simulink model "Demo_veDYNA_cs"  (Simulink 7.6)
settings: Solver=ode1  SolverMode=SingleTasking  StartTime=0  StopTime=15  FixedStep=1/500  RelTol=1e-3
PreLoadFcn:
  | PreScanveDYNAPreLoadFcn(bdroot);
  | check_NUTS_defined;
  | 
  | assignin('base',['model_closed_' bdroot],false);
PostLoadFcn:
  | PreScanveDYNAPostLoadFcn(bdroot);
  | 
InitFcn:
  | vdy_SetExternalInputSource('ManLongCtrl',1,'Brake','other');
  | vdy_SetExternalInputSource('ManLongCtrl',1,'EngineTorque','other');
  | vdy_SetExternalInputSource('ManLatCtrl',1,'Steering','other');
  | 
  | PreScanveDYNAInitFcn(bdroot);
  | PreScanExperimentInitFcn(bdroot)
StopFcn:
  | PreScanExperimentStopFcn(bdroot)
undefined symbols (not defined in the file): at_period, CPT, DiscIntNeverNeededParam, vm_at_pulsewidth, vm_driver_dflt_gain, x_ini_VRML, y_ini_VRML, z_ini_VRML
libraries: dyna_cpt_lib x93, PreScanSimulinkLibrary x10, PreScanUsefulBlocks x4, simulink x4, anilib x3, dyna_lib x3, simulink_extras x2, dyna_manctrl_lib x2, dyna_road_lib x2, dyna_io_lib x1, dyna_demo_lib x1, dyna_usr_maneuver_states_lib x1
(part 7 of 8)

== system Demo_veDYNA_cs/Vedyna_Vehicle/CPT_MDL/MDL_PAR/ManLongCtrl/System Instance 1/AccelerationY [m/s**2] ==
  Table : Lookup  InputValues=CPT.MDL_PAR.ManLongCtrl{1}.AccelerationY.Table.x  Table=CPT.MDL_PAR.ManLongCtrl{1}.AccelerationY.Table.v  SaturateOnIntegerOverflow=on
  Terminator : Terminator
  Terminator1 : Terminator
  Value : Constant  Value=CPT.MDL_PAR.ManLongCtrl{1}.AccelerationY.Value.v
  tag scope: ManLongCtrl_1_AccelerationY_TBL=global, ManLongCtrl_1_AccelerationY_VAL=global
  wires:
  [vdy_Simctrl_tsim] -> Table/1
  Value/1 -> [ManLongCtrl_1_AccelerationY_VAL]
  [ManLongCtrl_1_AccelerationY_VAL] -> Terminator/1
  [ManLongCtrl_1_AccelerationY_TBL] -> Terminator1/1
  Table/1 -> [ManLongCtrl_1_AccelerationY_TBL]

== system Demo_veDYNA_cs/Vedyna_Vehicle/CPT_MDL/MDL_PAR/ManLongCtrl/System Instance 1/Brake [%] ==
  Table : Lookup  InputValues=CPT.MDL_PAR.ManLongCtrl{1}.Brake.Table.x  Table=CPT.MDL_PAR.ManLongCtrl{1}.Brake.Table.v  SaturateOnIntegerOverflow=on
  Terminator : Terminator
  Terminator1 : Terminator
  Value : Constant  Value=CPT.MDL_PAR.ManLongCtrl{1}.Brake.Value.v
  tag scope: ManLongCtrl_1_Brake_TBL=global, ManLongCtrl_1_Brake_VAL=global
  wires:
  [vdy_Simctrl_tsim] -> Table/1
  Value/1 -> [ManLongCtrl_1_Brake_VAL]
  [ManLongCtrl_1_Brake_VAL] -> Terminator/1
  [ManLongCtrl_1_Brake_TBL] -> Terminator1/1
  Table/1 -> [ManLongCtrl_1_Brake_TBL]

== system Demo_veDYNA_cs/Vedyna_Vehicle/CPT_MDL/MDL_PAR/ManLongCtrl/System Instance 1/EngineTorque [Nm] ==
  Table : Lookup  InputValues=CPT.MDL_PAR.ManLongCtrl{1}.EngineTorque.Table.x  Table=CPT.MDL_PAR.ManLongCtrl{1}.EngineTorque.Table.v  SaturateOnIntegerOverflow=on
  Terminator : Terminator
  Terminator1 : Terminator
  Value : Constant  Value=CPT.MDL_PAR.ManLongCtrl{1}.EngineTorque.Value.v
  tag scope: ManLongCtrl_1_EngineTorque_TBL=global, ManLongCtrl_1_EngineTorque_VAL=global
  wires:
  [vdy_Simctrl_tsim] -> Table/1
  Value/1 -> [ManLongCtrl_1_EngineTorque_VAL]
  [ManLongCtrl_1_EngineTorque_VAL] -> Terminator/1
  [ManLongCtrl_1_EngineTorque_TBL] -> Terminator1/1
  Table/1 -> [ManLongCtrl_1_EngineTorque_TBL]

== system Demo_veDYNA_cs/Vedyna_Vehicle/CPT_MDL/MDL_PAR/ManLongCtrl/System Instance 1/Speed [km/h] ==
  Table : Lookup  InputValues=CPT.MDL_PAR.ManLongCtrl{1}.Speed.Table.x  Table=CPT.MDL_PAR.ManLongCtrl{1}.Speed.Table.v  SaturateOnIntegerOverflow=on
  Terminator : Terminator
  Terminator1 : Terminator
  Value : Constant  Value=CPT.MDL_PAR.ManLongCtrl{1}.Speed.Value.v
  tag scope: ManLongCtrl_1_Speed_TBL=global, ManLongCtrl_1_Speed_VAL=global
  wires:
  [vdy_Simctrl_tsim] -> Table/1
  Value/1 -> [ManLongCtrl_1_Speed_VAL]
  [ManLongCtrl_1_Speed_VAL] -> Terminator/1
  [ManLongCtrl_1_Speed_TBL] -> Terminator1/1
  Table/1 -> [ManLongCtrl_1_Speed_TBL]

== system Demo_veDYNA_cs/Vedyna_Vehicle/CPT_MDL/MDL_PAR/ManLongCtrl/System Instance 1/Throttle [%] ==
  Table : Lookup  InputValues=CPT.MDL_PAR.ManLongCtrl{1}.Throttle.Table.x  Table=CPT.MDL_PAR.ManLongCtrl{1}.Throttle.Table.v  SaturateOnIntegerOverflow=on
  Terminator : Terminator
  Terminator1 : Terminator
  Value : Constant  Value=CPT.MDL_PAR.ManLongCtrl{1}.Throttle.Value.v
  tag scope: ManLongCtrl_1_Throttle_TBL=global, ManLongCtrl_1_Throttle_VAL=global
  wires:
  [vdy_Simctrl_tsim] -> Table/1
  Value/1 -> [ManLongCtrl_1_Throttle_VAL]
  [ManLongCtrl_1_Throttle_VAL] -> Terminator/1
  [ManLongCtrl_1_Throttle_TBL] -> Terminator1/1
  Table/1 -> [ManLongCtrl_1_Throttle_TBL]

== system Demo_veDYNA_cs/Vedyna_Vehicle/CPT_MDL/MDL_PAR/Tmeasy/System Instance 1/RoadMueScale [0..1] ==
  Table : Lookup  InputValues=CPT.MDL_PAR.Tmeasy{1}.RoadMueScale.Table.x  Table=CPT.MDL_PAR.Tmeasy{1}.RoadMueScale.Table.v  SaturateOnIntegerOverflow=on
  Terminator : Terminator
  Terminator1 : Terminator
  Value : Constant  Value=CPT.MDL_PAR.Tmeasy{1}.RoadMueScale.Value.v
  tag scope: Tmeasy_1_RoadMueScale_TBL=global, Tmeasy_1_RoadMueScale_VAL=global
  wires:
  [vdy_Simctrl_tsim] -> Table/1
  Value/1 -> [Tmeasy_1_RoadMueScale_VAL]
  [Tmeasy_1_RoadMueScale_VAL] -> Terminator/1
  [Tmeasy_1_RoadMueScale_TBL] -> Terminator1/1
  Table/1 -> [Tmeasy_1_RoadMueScale_TBL]

== system Demo_veDYNA_cs/Vedyna_Vehicle/CPT_MDL/MDL_PAR/Tmeasy/System Instance 2/RoadMueScale [0..1] ==
  Table : Lookup  InputValues=CPT.MDL_PAR.Tmeasy{2}.RoadMueScale.Table.x  Table=CPT.MDL_PAR.Tmeasy{2}.RoadMueScale.Table.v  SaturateOnIntegerOverflow=on
  Terminator : Terminator
  Terminator1 : Terminator
  Value : Constant  Value=CPT.MDL_PAR.Tmeasy{2}.RoadMueScale.Value.v
  tag scope: Tmeasy_2_RoadMueScale_TBL=global, Tmeasy_2_RoadMueScale_VAL=global
  wires:
  [vdy_Simctrl_tsim] -> Table/1
  Value/1 -> [Tmeasy_2_RoadMueScale_VAL]
  [Tmeasy_2_RoadMueScale_VAL] -> Terminator/1
  [Tmeasy_2_RoadMueScale_TBL] -> Terminator1/1
  Table/1 -> [Tmeasy_2_RoadMueScale_TBL]

== system Demo_veDYNA_cs/Vedyna_Vehicle/CPT_MDL/MDL_PAR/Tmeasy/System Instance 3/RoadMueScale [0..1] ==
  Table : Lookup  InputValues=CPT.MDL_PAR.Tmeasy{3}.RoadMueScale.Table.x  Table=CPT.MDL_PAR.Tmeasy{3}.RoadMueScale.Table.v  SaturateOnIntegerOverflow=on
  Terminator : Terminator
  Terminator1 : Terminator
  Value : Constant  Value=CPT.MDL_PAR.Tmeasy{3}.RoadMueScale.Value.v
  tag scope: Tmeasy_3_RoadMueScale_TBL=global, Tmeasy_3_RoadMueScale_VAL=global
  wires:
  [vdy_Simctrl_tsim] -> Table/1
  Value/1 -> [Tmeasy_3_RoadMueScale_VAL]
  [Tmeasy_3_RoadMueScale_VAL] -> Terminator/1
  [Tmeasy_3_RoadMueScale_TBL] -> Terminator1/1
  Table/1 -> [Tmeasy_3_RoadMueScale_TBL]

== system Demo_veDYNA_cs/Vedyna_Vehicle/CPT_MDL/MDL_PAR/Tmeasy/System Instance 4/RoadMueScale [0..1] ==
  Table : Lookup  InputValues=CPT.MDL_PAR.Tmeasy{4}.RoadMueScale.Table.x  Table=CPT.MDL_PAR.Tmeasy{4}.RoadMueScale.Table.v  SaturateOnIntegerOverflow=on
  Terminator : Terminator
  Terminator1 : Terminator
  Value : Constant  Value=CPT.MDL_PAR.Tmeasy{4}.RoadMueScale.Value.v
  tag scope: Tmeasy_4_RoadMueScale_TBL=global, Tmeasy_4_RoadMueScale_VAL=global
  wires:
  [vdy_Simctrl_tsim] -> Table/1
  Value/1 -> [Tmeasy_4_RoadMueScale_VAL]
  [Tmeasy_4_RoadMueScale_VAL] -> Terminator/1
  [Tmeasy_4_RoadMueScale_TBL] -> Terminator1/1
  Table/1 -> [Tmeasy_4_RoadMueScale_TBL]

== system Demo_veDYNA_cs/Vedyna_Vehicle/CPT_MDL/MDL_PAR/Tmeasy/System Instance 5/RoadMueScale [0..1] ==
  Table : Lookup  InputValues=CPT.MDL_PAR.Tmeasy{5}.RoadMueScale.Table.x  Table=CPT.MDL_PAR.Tmeasy{5}.RoadMueScale.Table.v  SaturateOnIntegerOverflow=on
  Terminator : Terminator
  Terminator1 : Terminator
  Value : Constant  Value=CPT.MDL_PAR.Tmeasy{5}.RoadMueScale.Value.v
  tag scope: Tmeasy_5_RoadMueScale_TBL=global, Tmeasy_5_RoadMueScale_VAL=global
  wires:
  [vdy_Simctrl_tsim] -> Table/1
  Value/1 -> [Tmeasy_5_RoadMueScale_VAL]
  [Tmeasy_5_RoadMueScale_VAL] -> Terminator/1
  [Tmeasy_5_RoadMueScale_TBL] -> Terminator1/1
  Table/1 -> [Tmeasy_5_RoadMueScale_TBL]

== system Demo_veDYNA_cs/Vedyna_Vehicle/CPT_MDL/MDL_PAR/Tmeasy/System Instance 6/RoadMueScale [0..1] ==
  Table : Lookup  InputValues=CPT.MDL_PAR.Tmeasy{6}.RoadMueScale.Table.x  Table=CPT.MDL_PAR.Tmeasy{6}.RoadMueScale.Table.v  SaturateOnIntegerOverflow=on
  Terminator : Terminator
  Terminator1 : Terminator
  Value : Constant  Value=CPT.MDL_PAR.Tmeasy{6}.RoadMueScale.Value.v
  tag scope: Tmeasy_6_RoadMueScale_TBL=global, Tmeasy_6_RoadMueScale_VAL=global
  wires:
  [vdy_Simctrl_tsim] -> Table/1
  Value/1 -> [Tmeasy_6_RoadMueScale_VAL]
  [Tmeasy_6_RoadMueScale_VAL] -> Terminator/1
  [Tmeasy_6_RoadMueScale_TBL] -> Terminator1/1
  Table/1 -> [Tmeasy_6_RoadMueScale_TBL]

== system Demo_veDYNA_cs/Vedyna_Vehicle/CPT_MDL/MDL_PAR/Tmeasy/System Instance 7/RoadMueScale [0..1] ==
  Table : Lookup  InputValues=CPT.MDL_PAR.Tmeasy{7}.RoadMueScale.Table.x  Table=CPT.MDL_PAR.Tmeasy{7}.RoadMueScale.Table.v  SaturateOnIntegerOverflow=on
  Terminator : Terminator
  Terminator1 : Terminator
  Value : Constant  Value=CPT.MDL_PAR.Tmeasy{7}.RoadMueScale.Value.v
  tag scope: Tmeasy_7_RoadMueScale_TBL=global, Tmeasy_7_RoadMueScale_VAL=global
  wires:
  Table/1 -> [Tmeasy_7_RoadMueScale_TBL]
  [Tmeasy_7_RoadMueScale_TBL] -> Terminator1/1
  [Tmeasy_7_RoadMueScale_VAL] -> Terminator/1
  Value/1 -> [Tmeasy_7_RoadMueScale_VAL]
  [vdy_Simctrl_tsim] -> Table/1

== system Demo_veDYNA_cs/Vedyna_Vehicle/CPT_MDL/MDL_PAR/Tmeasy/System Instance 8/RoadMueScale [0..1] ==
  Table : Lookup  InputValues=CPT.MDL_PAR.Tmeasy{8}.RoadMueScale.Table.x  Table=CPT.MDL_PAR.Tmeasy{8}.RoadMueScale.Table.v  SaturateOnIntegerOverflow=on
  Terminator : Terminator
  Terminator1 : Terminator
  Value : Constant  Value=CPT.MDL_PAR.Tmeasy{8}.RoadMueScale.Value.v
  tag scope: Tmeasy_8_RoadMueScale_TBL=global, Tmeasy_8_RoadMueScale_VAL=global
  wires:
  Table/1 -> [Tmeasy_8_RoadMueScale_TBL]
  [Tmeasy_8_RoadMueScale_TBL] -> Terminator1/1
  [Tmeasy_8_RoadMueScale_VAL] -> Terminator/1
  Value/1 -> [Tmeasy_8_RoadMueScale_VAL]
  [vdy_Simctrl_tsim] -> Table/1

== system Demo_veDYNA_cs/Vedyna_Vehicle/CPT_MDL/MDL_PAR/Wheel/System Instance 1/pbrm [N/m**2] ==
  Table : Lookup  InputValues=CPT.MDL_PAR.Wheel{1}.pbrm.Table.x  Table=CPT.MDL_PAR.Wheel{1}.pbrm.Table.v  SaturateOnIntegerOverflow=on
  Terminator : Terminator
  Terminator1 : Terminator
  Value : Constant  Value=CPT.MDL_PAR.Wheel{1}.pbrm.Value.v
  tag scope: Wheel_1_pbrm_TBL=global, Wheel_1_pbrm_VAL=global
  wires:
  [vdy_Simctrl_tsim] -> Table/1
  Value/1 -> [Wheel_1_pbrm_VAL]
  [Wheel_1_pbrm_VAL] -> Terminator/1
  [Wheel_1_pbrm_TBL] -> Terminator1/1
  Table/1 -> [Wheel_1_pbrm_TBL]

== system Demo_veDYNA_cs/Vedyna_Vehicle/CPT_MDL/MDL_PAR/Wheel/System Instance 2/pbrm [N/m**2] ==
  Table : Lookup  InputValues=CPT.MDL_PAR.Wheel{2}.pbrm.Table.x  Table=CPT.MDL_PAR.Wheel{2}.pbrm.Table.v  SaturateOnIntegerOverflow=on
  Terminator : Terminator
  Terminator1 : Terminator
  Value : Constant  Value=CPT.MDL_PAR.Wheel{2}.pbrm.Value.v
  tag scope: Wheel_2_pbrm_TBL=global, Wheel_2_pbrm_VAL=global
  wires:
  [vdy_Simctrl_tsim] -> Table/1
  Value/1 -> [Wheel_2_pbrm_VAL]
  [Wheel_2_pbrm_VAL] -> Terminator/1
  [Wheel_2_pbrm_TBL] -> Terminator1/1
  Table/1 -> [Wheel_2_pbrm_TBL]

== system Demo_veDYNA_cs/Vedyna_Vehicle/CPT_MDL/MDL_PAR/Wheel/System Instance 3/pbrm [N/m**2] ==
  Table : Lookup  InputValues=CPT.MDL_PAR.Wheel{3}.pbrm.Table.x  Table=CPT.MDL_PAR.Wheel{3}.pbrm.Table.v  SaturateOnIntegerOverflow=on
  Terminator : Terminator
  Terminator1 : Terminator
  Value : Constant  Value=CPT.MDL_PAR.Wheel{3}.pbrm.Value.v
  tag scope: Wheel_3_pbrm_TBL=global, Wheel_3_pbrm_VAL=global
  wires:
  [vdy_Simctrl_tsim] -> Table/1
  Value/1 -> [Wheel_3_pbrm_VAL]
  [Wheel_3_pbrm_VAL] -> Terminator/1
  [Wheel_3_pbrm_TBL] -> Terminator1/1
  Table/1 -> [Wheel_3_pbrm_TBL]

== system Demo_veDYNA_cs/Vedyna_Vehicle/CPT_MDL/MDL_PAR/Wheel/System Instance 4/pbrm [N/m**2] ==
  Table : Lookup  InputValues=CPT.MDL_PAR.Wheel{4}.pbrm.Table.x  Table=CPT.MDL_PAR.Wheel{4}.pbrm.Table.v  SaturateOnIntegerOverflow=on
  Terminator : Terminator
  Terminator1 : Terminator
  Value : Constant  Value=CPT.MDL_PAR.Wheel{4}.pbrm.Value.v
  tag scope: Wheel_4_pbrm_TBL=global, Wheel_4_pbrm_VAL=global
  wires:
  [vdy_Simctrl_tsim] -> Table/1
  Value/1 -> [Wheel_4_pbrm_VAL]
  [Wheel_4_pbrm_VAL] -> Terminator/1
  [Wheel_4_pbrm_TBL] -> Terminator1/1
  Table/1 -> [Wheel_4_pbrm_TBL]

== system Demo_veDYNA_cs/Vedyna_Vehicle/CPT_MDL/MDL_PAR/Wheel/System Instance 5/pbrm [N/m**2] ==
  Table : Lookup  InputValues=CPT.MDL_PAR.Wheel{5}.pbrm.Table.x  Table=CPT.MDL_PAR.Wheel{5}.pbrm.Table.v  SaturateOnIntegerOverflow=on
  Terminator : Terminator
  Terminator1 : Terminator
  Value : Constant  Value=CPT.MDL_PAR.Wheel{5}.pbrm.Value.v
  tag scope: Wheel_5_pbrm_TBL=global, Wheel_5_pbrm_VAL=global
  wires:
  [vdy_Simctrl_tsim] -> Table/1
  Value/1 -> [Wheel_5_pbrm_VAL]
  [Wheel_5_pbrm_VAL] -> Terminator/1
  [Wheel_5_pbrm_TBL] -> Terminator1/1
  Table/1 -> [Wheel_5_pbrm_TBL]

== system Demo_veDYNA_cs/Vedyna_Vehicle/CPT_MDL/MDL_PAR/Wheel/System Instance 6/pbrm [N/m**2] ==
  Table : Lookup  InputValues=CPT.MDL_PAR.Wheel{6}.pbrm.Table.x  Table=CPT.MDL_PAR.Wheel{6}.pbrm.Table.v  SaturateOnIntegerOverflow=on
  Terminator : Terminator
  Terminator1 : Terminator
  Value : Constant  Value=CPT.MDL_PAR.Wheel{6}.pbrm.Value.v
  tag scope: Wheel_6_pbrm_TBL=global, Wheel_6_pbrm_VAL=global
  wires:
  [vdy_Simctrl_tsim] -> Table/1
  Value/1 -> [Wheel_6_pbrm_VAL]
  [Wheel_6_pbrm_VAL] -> Terminator/1
  [Wheel_6_pbrm_TBL] -> Terminator1/1
  Table/1 -> [Wheel_6_pbrm_TBL]

== system Demo_veDYNA_cs/Vedyna_Vehicle/CPT_MDL/MDL_PAR/Wheel/System Instance 7/pbrm [N/m**2] ==
  Table : Lookup  InputValues=CPT.MDL_PAR.Wheel{7}.pbrm.Table.x  Table=CPT.MDL_PAR.Wheel{7}.pbrm.Table.v  SaturateOnIntegerOverflow=on
  Terminator : Terminator
  Terminator1 : Terminator
  Value : Constant  Value=CPT.MDL_PAR.Wheel{7}.pbrm.Value.v
  tag scope: Wheel_7_pbrm_TBL=global, Wheel_7_pbrm_VAL=global
  wires:
  Table/1 -> [Wheel_7_pbrm_TBL]
  [Wheel_7_pbrm_TBL] -> Terminator1/1
  [Wheel_7_pbrm_VAL] -> Terminator/1
  Value/1 -> [Wheel_7_pbrm_VAL]
  [vdy_Simctrl_tsim] -> Table/1

== system Demo_veDYNA_cs/Vedyna_Vehicle/CPT_MDL/MDL_PAR/Wheel/System Instance 8/pbrm [N/m**2] ==
  Table : Lookup  InputValues=CPT.MDL_PAR.Wheel{8}.pbrm.Table.x  Table=CPT.MDL_PAR.Wheel{8}.pbrm.Table.v  SaturateOnIntegerOverflow=on
  Terminator : Terminator
  Terminator1 : Terminator
  Value : Constant  Value=CPT.MDL_PAR.Wheel{8}.pbrm.Value.v
  tag scope: Wheel_8_pbrm_TBL=global, Wheel_8_pbrm_VAL=global
  wires:
  Table/1 -> [Wheel_8_pbrm_TBL]
  [Wheel_8_pbrm_TBL] -> Terminator1/1
  [Wheel_8_pbrm_VAL] -> Terminator/1
  Value/1 -> [Wheel_8_pbrm_VAL]
  [vdy_Simctrl_tsim] -> Table/1

== system Demo_veDYNA_cs/Vedyna_Vehicle/CPT_MDL/MDL_SW/BrkHyd/System Instance 1/HCI [1,..,n] ==
  Switch : Constant  Value=CPT.MDL_SW.BrkHyd{1}.HCI.Switch.v
  Terminator : Terminator
  tag scope: BrkHyd_1_HCI_SW=global
  wires:
  [BrkHyd_1_HCI_SW] -> Terminator/1
  Switch/1 -> [BrkHyd_1_HCI_SW]

== system Demo_veDYNA_cs/Vedyna_Vehicle/CPT_MDL/MDL_SW/BrkHyd/System Instance 1/pbrmaster [1,..,4] ==
  Switch : Constant  Value=CPT.MDL_SW.BrkHyd{1}.pbrmaster.Switch.v
  Terminator : Terminator
  tag scope: BrkHyd_1_pbrmaster_SW=global
  wires:
  [BrkHyd_1_pbrmaster_SW] -> Terminator/1
  Switch/1 -> [BrkHyd_1_pbrmaster_SW]

== system Demo_veDYNA_cs/Vedyna_Vehicle/CPT_MDL/MDL_SW/Chassis/System Instance 1/HCI [1,..,n] ==
  Switch : Constant  Value=CPT.MDL_SW.Chassis{1}.HCI.Switch.v
  Terminator : Terminator
  tag scope: Chassis_1_HCI_SW=global
  wires:
  [Chassis_1_HCI_SW] -> Terminator/1
  Switch/1 -> [Chassis_1_HCI_SW]

== system Demo_veDYNA_cs/Vedyna_Vehicle/CPT_MDL/MDL_SW/ClutchCtrl/System Instance 1/Clutch [1,..,4] ==
  Switch : Constant  Value=CPT.MDL_SW.ClutchCtrl{1}.Clutch.Switch.v
  Terminator : Terminator
  tag scope: ClutchCtrl_1_Clutch_SW=global
  wires:
  [ClutchCtrl_1_Clutch_SW] -> Terminator/1
  Switch/1 -> [ClutchCtrl_1_Clutch_SW]

== system Demo_veDYNA_cs/Vedyna_Vehicle/CPT_MDL/MDL_SW/ClutchCtrl/System Instance 1/ClutchMode [0,1] ==
  Switch : Constant  Value=CPT.MDL_SW.ClutchCtrl{1}.ClutchMode.Switch.v
  Terminator : Terminator
  tag scope: ClutchCtrl_1_ClutchMode_SW=global
  wires:
  [ClutchCtrl_1_ClutchMode_SW] -> Terminator/1
  Switch/1 -> [ClutchCtrl_1_ClutchMode_SW]

== system Demo_veDYNA_cs/Vedyna_Vehicle/CPT_MDL/MDL_SW/ClutchCtrl/System Instance 1/HCI [1,..,n] ==
  Switch : Constant  Value=CPT.MDL_SW.ClutchCtrl{1}.HCI.Switch.v
  Terminator : Terminator
  tag scope: ClutchCtrl_1_HCI_SW=global
  wires:
  [ClutchCtrl_1_HCI_SW] -> Terminator/1
  Switch/1 -> [ClutchCtrl_1_HCI_SW]

== system Demo_veDYNA_cs/Vedyna_Vehicle/CPT_MDL/MDL_SW/Contact/System Instance 1/RoadZ [1,..,4] ==
  Switch : Constant  Value=CPT.MDL_SW.Contact{1}.RoadZ.Switch.v
  Terminator : Terminator
  tag scope: Contact_1_RoadZ_SW=global
  wires:
  [Contact_1_RoadZ_SW] -> Terminator/1
  Switch/1 -> [Contact_1_RoadZ_SW]

== system Demo_veDYNA_cs/Vedyna_Vehicle/CPT_MDL/MDL_SW/Contact/System Instance 2/RoadZ [1,..,4] ==
  Switch : Constant  Value=CPT.MDL_SW.Contact{2}.RoadZ.Switch.v
  Terminator : Terminator
  tag scope: Contact_2_RoadZ_SW=global
  wires:
  [Contact_2_RoadZ_SW] -> Terminator/1
  Switch/1 -> [Contact_2_RoadZ_SW]

== system Demo_veDYNA_cs/Vedyna_Vehicle/CPT_MDL/MDL_SW/Contact/System Instance 3/RoadZ [1,..,4] ==
  Switch : Constant  Value=CPT.MDL_SW.Contact{3}.RoadZ.Switch.v
  Terminator : Terminator
  tag scope: Contact_3_RoadZ_SW=global
  wires:
  [Contact_3_RoadZ_SW] -> Terminator/1
  Switch/1 -> [Contact_3_RoadZ_SW]

== system Demo_veDYNA_cs/Vedyna_Vehicle/CPT_MDL/MDL_SW/Contact/System Instance 4/RoadZ [1,..,4] ==
  Switch : Constant  Value=CPT.MDL_SW.Contact{4}.RoadZ.Switch.v
  Terminator : Terminator
  tag scope: Contact_4_RoadZ_SW=global
  wires:
  [Contact_4_RoadZ_SW] -> Terminator/1
  Switch/1 -> [Contact_4_RoadZ_SW]

== system Demo_veDYNA_cs/Vedyna_Vehicle/CPT_MDL/MDL_SW/Contact/System Instance 5/RoadZ [1,..,4] ==
  Switch : Constant  Value=CPT.MDL_SW.Contact{5}.RoadZ.Switch.v
  Terminator : Terminator
  tag scope: Contact_5_RoadZ_SW=global
  wires:
  [Contact_5_RoadZ_SW] -> Terminator/1
  Switch/1 -> [Contact_5_RoadZ_SW]

== system Demo_veDYNA_cs/Vedyna_Vehicle/CPT_MDL/MDL_SW/Contact/System Instance 6/RoadZ [1,..,4] ==
  Switch : Constant  Value=CPT.MDL_SW.Contact{6}.RoadZ.Switch.v
  Terminator : Terminator
  tag scope: Contact_6_RoadZ_SW=global
  wires:
  [Contact_6_RoadZ_SW] -> Terminator/1
  Switch/1 -> [Contact_6_RoadZ_SW]

== system Demo_veDYNA_cs/Vedyna_Vehicle/CPT_MDL/MDL_SW/Contact/System Instance 7/RoadZ [1,..,4] ==
  Switch : Constant  Value=CPT.MDL_SW.Contact{7}.RoadZ.Switch.v
  Terminator : Terminator
  tag scope: Contact_7_RoadZ_SW=global
  wires:
  Switch/1 -> [Contact_7_RoadZ_SW]
  [Contact_7_RoadZ_SW] -> Terminator/1

== system Demo_veDYNA_cs/Vedyna_Vehicle/CPT_MDL/MDL_SW/Contact/System Instance 8/RoadZ [1,..,4] ==
  Switch : Constant  Value=CPT.MDL_SW.Contact{8}.RoadZ.Switch.v
  Terminator : Terminator
  tag scope: Contact_8_RoadZ_SW=global
  wires:
  Switch/1 -> [Contact_8_RoadZ_SW]
  [Contact_8_RoadZ_SW] -> Terminator/1

== system Demo_veDYNA_cs/Vedyna_Vehicle/CPT_MDL/MDL_SW/Driveline/System Instance 1/HCI [1,..,n] ==
  Switch : Constant  Value=CPT.MDL_SW.Driveline{1}.HCI.Switch.v
  Terminator : Terminator
  tag scope: Driveline_1_HCI_SW=global
  wires:
  [Driveline_1_HCI_SW] -> Terminator/1
  Switch/1 -> [Driveline_1_HCI_SW]

== system Demo_veDYNA_cs/Vedyna_Vehicle/CPT_MDL/MDL_SW/Driver/System Instance 1/HCI [1,..,n] ==
  Switch : Constant  Value=CPT.MDL_SW.Driver{1}.HCI.Switch.v
  Terminator : Terminator
  tag scope: Driver_1_HCI_SW=global
  wires:
  [Driver_1_HCI_SW] -> Terminator/1
  Switch/1 -> [Driver_1_HCI_SW]

== system Demo_veDYNA_cs/Vedyna_Vehicle/CPT_MDL/MDL_SW/Driver/System Instance 1/acc_comp_scale [1,..,4] ==
  Switch : Constant  Value=CPT.MDL_SW.Driver{1}.acc_comp_scale.Switch.v
  Terminator : Terminator
  tag scope: Driver_1_acc_comp_scale_SW=global
  wires:
  [Driver_1_acc_comp_scale_SW] -> Terminator/1
  Switch/1 -> [Driver_1_acc_comp_scale_SW]

== system Demo_veDYNA_cs/Vedyna_Vehicle/CPT_MDL/MDL_SW/Driver/System Instance 1/adj_acc_gain [1,..,4] ==
  Switch : Constant  Value=CPT.MDL_SW.Driver{1}.adj_acc_gain.Switch.v
  Terminator : Terminator
  tag scope: Driver_1_adj_acc_gain_SW=global
  wires:
  [Driver_1_adj_acc_gain_SW] -> Terminator/1
  Switch/1 -> [Driver_1_adj_acc_gain_SW]

== system Demo_veDYNA_cs/Vedyna_Vehicle/CPT_MDL/MDL_SW/Driver/System Instance 1/adj_brake_gain [1,..,4] ==
  Switch : Constant  Value=CPT.MDL_SW.Driver{1}.adj_brake_gain.Switch.v
  Terminator : Terminator
  tag scope: Driver_1_adj_brake_gain_SW=global
  wires:
  [Driver_1_adj_brake_gain_SW] -> Terminator/1
  Switch/1 -> [Driver_1_adj_brake_gain_SW]

== system Demo_veDYNA_cs/Vedyna_Vehicle/CPT_MDL/MDL_SW/Driver/System Instance 1/ax_min [1,..,4] ==
  Switch : Constant  Value=CPT.MDL_SW.Driver{1}.ax_min.Switch.v
  Terminator : Terminator
  tag scope: Driver_1_ax_min_SW=global
  wires:
  [Driver_1_ax_min_SW] -> Terminator/1
  Switch/1 -> [Driver_1_ax_min_SW]

== system Demo_veDYNA_cs/Vedyna_Vehicle/CPT_MDL/MDL_SW/Driver/System Instance 1/ctrl_acc_smooth_t [1,..,4] ==
  Switch : Constant  Value=CPT.MDL_SW.Driver{1}.ctrl_acc_smooth_t.Switch.v
  Terminator : Terminator
  tag scope: Driver_1_ctrl_acc_smooth_t_SW=global
  wires:
  [Driver_1_ctrl_acc_smooth_t_SW] -> Terminator/1
  Switch/1 -> [Driver_1_ctrl_acc_smooth_t_SW]

== system Demo_veDYNA_cs/Vedyna_Vehicle/CPT_MDL/MDL_SW/Driver/System Instance 1/cu_comp_scale [1,..,4] ==
  Switch : Constant  Value=CPT.MDL_SW.Driver{1}.cu_comp_scale.Switch.v
  Terminator : Terminator
  tag scope: Driver_1_cu_comp_scale_SW=global
  wires:
  [Driver_1_cu_comp_scale_SW] -> Terminator/1
  Switch/1 -> [Driver_1_cu_comp_scale_SW]

== system Demo_veDYNA_cs/Vedyna_Vehicle/CPT_MDL/MDL_SW/Driver/System Instance 1/cu_path [1,..,4] ==
  Switch : Constant  Value=CPT.MDL_SW.Driver{1}.cu_path.Switch.v
  Terminator : Terminator
  tag scope: Driver_1_cu_path_SW=global
  wires:
  [Driver_1_cu_path_SW] -> Terminator/1
  Switch/1 -> [Driver_1_cu_path_SW]

== system Demo_veDYNA_cs/Vedyna_Vehicle/CPT_MDL/MDL_SW/Driver/System Instance 1/front_stiff [1,..,4] ==
  Switch : Constant  Value=CPT.MDL_SW.Driver{1}.front_stiff.Switch.v
  Terminator : Terminator
  tag scope: Driver_1_front_stiff_SW=global
  wires:
  [Driver_1_front_stiff_SW] -> Terminator/1
  Switch/1 -> [Driver_1_front_stiff_SW]

== system Demo_veDYNA_cs/Vedyna_Vehicle/CPT_MDL/MDL_SW/Driver/System Instance 1/front_stiff_sw [1,..,4] ==
  Switch : Constant  Value=CPT.MDL_SW.Driver{1}.front_stiff_sw.Switch.v
  Terminator : Terminator
  tag scope: Driver_1_front_stiff_sw_SW=global
  wires:
  [Driver_1_front_stiff_sw_SW] -> Terminator/1
  Switch/1 -> [Driver_1_front_stiff_sw_SW]

== system Demo_veDYNA_cs/Vedyna_Vehicle/CPT_MDL/MDL_SW/Driver/System Instance 1/gain_lat [1,..,4] ==
  Switch : Constant  Value=CPT.MDL_SW.Driver{1}.gain_lat.Switch.v
  Terminator : Terminator
  tag scope: Driver_1_gain_lat_SW=global
  wires:
  [Driver_1_gain_lat_SW] -> Terminator/1
  Switch/1 -> [Driver_1_gain_lat_SW]

== system Demo_veDYNA_cs/Vedyna_Vehicle/CPT_MDL/MDL_SW/Driver/System Instance 1/gain_long [1,..,4] ==
  Switch : Constant  Value=CPT.MDL_SW.Driver{1}.gain_long.Switch.v
  Terminator : Terminator
  tag scope: Driver_1_gain_long_SW=global
  wires:
  [Driver_1_gain_long_SW] -> Terminator/1
  Switch/1 -> [Driver_1_gain_long_SW]

== system Demo_veDYNA_cs/Vedyna_Vehicle/CPT_MDL/MDL_SW/Driver/System Instance 1/lat_for_r_scale [1,..,4] ==
  Switch : Constant  Value=CPT.MDL_SW.Driver{1}.lat_for_r_scale.Switch.v
  Terminator : Terminator
  tag scope: Driver_1_lat_for_r_scale_SW=global
  wires:
  [Driver_1_lat_for_r_scale_SW] -> Terminator/1
  Switch/1 -> [Driver_1_lat_for_r_scale_SW]

== system Demo_veDYNA_cs/Vedyna_Vehicle/CPT_MDL/MDL_SW/Driver/System Instance 1/lat_for_r_smooth_t [1,..,4] ==
  Switch : Constant  Value=CPT.MDL_SW.Driver{1}.lat_for_r_smooth_t.Switch.v
  Terminator : Terminator
  tag scope: Driver_1_lat_for_r_smooth_t_SW=global
  wires:
  [Driver_1_lat_for_r_smooth_t_SW] -> Terminator/1
  Switch/1 -> [Driver_1_lat_for_r_smooth_t_SW]

== system Demo_veDYNA_cs/Vedyna_Vehicle/CPT_MDL/MDL_SW/Driver/System Instance 1/lat_for_r_sw [1,..,4] ==
  Switch : Constant  Value=CPT.MDL_SW.Driver{1}.lat_for_r_sw.Switch.v
  Terminator : Terminator
  tag scope: Driver_1_lat_for_r_sw_SW=global
  wires:
  [Driver_1_lat_for_r_sw_SW] -> Terminator/1
  Switch/1 -> [Driver_1_lat_for_r_sw_SW]

== system Demo_veDYNA_cs/Vedyna_Vehicle/CPT_MDL/MDL_SW/Driver/System Instance 1/path_v_scale [1,..,4] ==
  Switch : Constant  Value=CPT.MDL_SW.Driver{1}.path_v_scale.Switch.v
  Terminator : Terminator
  tag scope: Driver_1_path_v_scale_SW=global
  wires:
  [Driver_1_path_v_scale_SW] -> Terminator/1
  Switch/1 -> [Driver_1_path_v_scale_SW]

== system Demo_veDYNA_cs/Vedyna_Vehicle/CPT_MDL/MDL_SW/Driver/System Instance 1/path_x_offset [1,..,4] ==
  Switch : Constant  Value=CPT.MDL_SW.Driver{1}.path_x_offset.Switch.v
  Terminator : Terminator
  tag scope: Driver_1_path_x_offset_SW=global
  wires:
  [Driver_1_path_x_offset_SW] -> Terminator/1
  Switch/1 -> [Driver_1_path_x_offset_SW]

== system Demo_veDYNA_cs/Vedyna_Vehicle/CPT_MDL/MDL_SW/Driver/System Instance 1/psi_path [1,..,4] ==
  Switch : Constant  Value=CPT.MDL_SW.Driver{1}.psi_path.Switch.v
  Terminator : Terminator
  tag scope: Driver_1_psi_path_SW=global
  wires:
  [Driver_1_psi_path_SW] -> Terminator/1
  Switch/1 -> [Driver_1_psi_path_SW]

== system Demo_veDYNA_cs/Vedyna_Vehicle/CPT_MDL/MDL_SW/Driver/System Instance 1/q_path [1,..,4] ==
  Switch : Constant  Value=CPT.MDL_SW.Driver{1}.q_path.Switch.v
  Terminator : Terminator
  tag scope: Driver_1_q_path_SW=global
  wires:
  [Driver_1_q_path_SW] -> Terminator/1
  Switch/1 -> [Driver_1_q_path_SW]

== system Demo_veDYNA_cs/Vedyna_Vehicle/CPT_MDL/MDL_SW/Driver/System Instance 1/rear_stiff [1,..,4] ==
  Switch : Constant  Value=CPT.MDL_SW.Driver{1}.rear_stiff.Switch.v
  Terminator : Terminator
  tag scope: Driver_1_rear_stiff_SW=global
  wires:
  [Driver_1_rear_stiff_SW] -> Terminator/1
  Switch/1 -> [Driver_1_rear_stiff_SW]

== system Demo_veDYNA_cs/Vedyna_Vehicle/CPT_MDL/MDL_SW/Driver/System Instance 1/rear_stiff_sw [1,..,4] ==
  Switch : Constant  Value=CPT.MDL_SW.Driver{1}.rear_stiff_sw.Switch.v
  Terminator : Terminator
  tag scope: Driver_1_rear_stiff_sw_SW=global
  wires:
  [Driver_1_rear_stiff_sw_SW] -> Terminator/1
  Switch/1 -> [Driver_1_rear_stiff_sw_SW]

== system Demo_veDYNA_cs/Vedyna_Vehicle/CPT_MDL/MDL_SW/Driver/System Instance 1/steer_max [1,..,4] ==
  Switch : Constant  Value=CPT.MDL_SW.Driver{1}.steer_max.Switch.v
  Terminator : Terminator
  tag scope: Driver_1_steer_max_SW=global
  wires:
  [Driver_1_steer_max_SW] -> Terminator/1
  Switch/1 -> [Driver_1_steer_max_SW]

== system Demo_veDYNA_cs/Vedyna_Vehicle/CPT_MDL/MDL_SW/Driver/System Instance 1/steer_min [1,..,4] ==
  Switch : Constant  Value=CPT.MDL_SW.Driver{1}.steer_min.Switch.v
  Terminator : Terminator
  tag scope: Driver_1_steer_min_SW=global
  wires:
  [Driver_1_steer_min_SW] -> Terminator/1
  Switch/1 -> [Driver_1_steer_min_SW]

== system Demo_veDYNA_cs/Vedyna_Vehicle/CPT_MDL/MDL_SW/Driver/System Instance 1/steer_rate_max [1,..,4] ==
  Switch : Constant  Value=CPT.MDL_SW.Driver{1}.steer_rate_max.Switch.v
  Terminator : Terminator
  tag scope: Driver_1_steer_rate_max_SW=global
  wires:
  [Driver_1_steer_rate_max_SW] -> Terminator/1
  Switch/1 -> [Driver_1_steer_rate_max_SW]

== system Demo_veDYNA_cs/Vedyna_Vehicle/CPT_MDL/MDL_SW/Driver/System Instance 1/steer_rate_min [1,..,4] ==
  Switch : Constant  Value=CPT.MDL_SW.Driver{1}.steer_rate_min.Switch.v
  Terminator : Terminator
  tag scope: Driver_1_steer_rate_min_SW=global
  wires:
  [Driver_1_steer_rate_min_SW] -> Terminator/1
  Switch/1 -> [Driver_1_steer_rate_min_SW]

== system Demo_veDYNA_cs/Vedyna_Vehicle/CPT_MDL/MDL_SW/Driver/System Instance 1/steer_smooth_t [1,..,4] ==
  Switch : Constant  Value=CPT.MDL_SW.Driver{1}.steer_smooth_t.Switch.v
  Terminator : Terminator
  tag scope: Driver_1_steer_smooth_t_SW=global
  wires:
  [Driver_1_steer_smooth_t_SW] -> Terminator/1
  Switch/1 -> [Driver_1_steer_smooth_t_SW]

== system Demo_veDYNA_cs/Vedyna_Vehicle/CPT_MDL/MDL_SW/Driver/System Instance 1/target_aim_x [1,..,4] ==
  Switch : Constant  Value=CPT.MDL_SW.Driver{1}.target_aim_x.Switch.v
  Terminator : Terminator
  tag scope: Driver_1_target_aim_x_SW=global
  wires:
  [Driver_1_target_aim_x_SW] -> Terminator/1
  Switch/1 -> [Driver_1_target_aim_x_SW]

== system Demo_veDYNA_cs/Vedyna_Vehicle/CPT_MDL/MDL_SW/Driver/System Instance 1/tgt_a_max [1,..,4] ==
  Switch : Constant  Value=CPT.MDL_SW.Driver{1}.tgt_a_max.Switch.v
  Terminator : Terminator
  tag scope: Driver_1_tgt_a_max_SW=global
  wires:
  [Driver_1_tgt_a_max_SW] -> Terminator/1
  Switch/1 -> [Driver_1_tgt_a_max_SW]

== system Demo_veDYNA_cs/Vedyna_Vehicle/CPT_MDL/MDL_SW/Driver/System Instance 1/tgt_acc_smooth_t [1,..,4] ==
  Switch : Constant  Value=CPT.MDL_SW.Driver{1}.tgt_acc_smooth_t.Switch.v
  Terminator : Terminator
  tag scope: Driver_1_tgt_acc_smooth_t_SW=global
  wires:
  [Driver_1_tgt_acc_smooth_t_SW] -> Terminator/1
  Switch/1 -> [Driver_1_tgt_acc_smooth_t_SW]

== system Demo_veDYNA_cs/Vedyna_Vehicle/CPT_MDL/MDL_SW/Driver/System Instance 1/tgt_ax_max [1,..,4] ==
  Switch : Constant  Value=CPT.MDL_SW.Driver{1}.tgt_ax_max.Switch.v
  Terminator : Terminator
  tag scope: Driver_1_tgt_ax_max_SW=global
  wires:
  [Driver_1_tgt_ax_max_SW] -> Terminator/1
  Switch/1 -> [Driver_1_tgt_ax_max_SW]

== system Demo_veDYNA_cs/Vedyna_Vehicle/CPT_MDL/MDL_SW/Driver/System Instance 1/tgt_ax_min [1,..,4] ==
  Switch : Constant  Value=CPT.MDL_SW.Driver{1}.tgt_ax_min.Switch.v
  Terminator : Terminator
  tag scope: Driver_1_tgt_ax_min_SW=global
  wires:
  [Driver_1_tgt_ax_min_SW] -> Terminator/1
  Switch/1 -> [Driver_1_tgt_ax_min_SW]

== system Demo_veDYNA_cs/Vedyna_Vehicle/CPT_MDL/MDL_SW/Driver/System Instance 1/tgt_ay_max [1,..,4] ==
  Switch : Constant  Value=CPT.MDL_SW.Driver{1}.tgt_ay_max.Switch.v
  Terminator : Terminator
  tag scope: Driver_1_tgt_ay_max_SW=global
  wires:
  [Driver_1_tgt_ay_max_SW] -> Terminator/1
  Switch/1 -> [Driver_1_tgt_ay_max_SW]

== system Demo_veDYNA_cs/Vedyna_Vehicle/CPT_MDL/MDL_SW/Driver/System Instance 1/tgt_v_max [1,..,4] ==
  Switch : Constant  Value=CPT.MDL_SW.Driver{1}.tgt_v_max.Switch.v
  Terminator : Terminator
  tag scope: Driver_1_tgt_v_max_SW=global
  wires:
  [Driver_1_tgt_v_max_SW] -> Terminator/1
  Switch/1 -> [Driver_1_tgt_v_max_SW]

== system Demo_veDYNA_cs/Vedyna_Vehicle/CPT_MDL/MDL_SW/Driver/System Instance 1/tgt_v_min [1,..,4] ==
  Switch : Constant  Value=CPT.MDL_SW.Driver{1}.tgt_v_min.Switch.v
  Terminator : Terminator
  tag scope: Driver_1_tgt_v_min_SW=global
  wires:
  [Driver_1_tgt_v_min_SW] -> Terminator/1
  Switch/1 -> [Driver_1_tgt_v_min_SW]

== system Demo_veDYNA_cs/Vedyna_Vehicle/CPT_MDL/MDL_SW/Driver/System Instance 1/use_simulink_sw [1,..,4] ==
  Switch : Constant  Value=CPT.MDL_SW.Driver{1}.use_simulink_sw.Switch.v
  Terminator : Terminator
  tag scope: Driver_1_use_simulink_sw_SW=global
  wires:
  [Driver_1_use_simulink_sw_SW] -> Terminator/1
  Switch/1 -> [Driver_1_use_simulink_sw_SW]

== system Demo_veDYNA_cs/Vedyna_Vehicle/CPT_MDL/MDL_SW/Driver/System Instance 1/v_comp_scale [1,..,4] ==
  Switch : Constant  Value=CPT.MDL_SW.Driver{1}.v_comp_scale.Switch.v
  Terminator : Terminator
  tag scope: Driver_1_v_comp_scale_SW=global
  wires:
  [Driver_1_v_comp_scale_SW] -> Terminator/1
  Switch/1 -> [Driver_1_v_comp_scale_SW]

== system Demo_veDYNA_cs/Vedyna_Vehicle/CPT_MDL/MDL_SW/Driver/System Instance 1/v_path [1,..,4] ==
  Switch : Constant  Value=CPT.MDL_SW.Driver{1}.v_path.Switch.v
  Terminator : Terminator
  tag scope: Driver_1_v_path_SW=global
  wires:
  [Driver_1_v_path_SW] -> Terminator/1
  Switch/1 -> [Driver_1_v_path_SW]

== system Demo_veDYNA_cs/Vedyna_Vehicle/CPT_MDL/MDL_SW/Engine/System Instance 1/ASR_Flag [1,..,4] ==
  Switch : Constant  Value=CPT.MDL_SW.Engine{1}.ASR_Flag.Switch.v
  Terminator : Terminator
  tag scope: Engine_1_ASR_Flag_SW=global
  wires:
  [Engine_1_ASR_Flag_SW] -> Terminator/1
  Switch/1 -> [Engine_1_ASR_Flag_SW]

== system Demo_veDYNA_cs/Vedyna_Vehicle/CPT_MDL/MDL_SW/Engine/System Instance 1/ASR_Torque [1,..,4] ==
  Switch : Constant  Value=CPT.MDL_SW.Engine{1}.ASR_Torque.Switch.v
  Terminator : Terminator
  tag scope: Engine_1_ASR_Torque_SW=global
  wires:
  [Engine_1_ASR_Torque_SW] -> Terminator/1
  Switch/1 -> [Engine_1_ASR_Torque_SW]

== system Demo_veDYNA_cs/Vedyna_Vehicle/CPT_MDL/MDL_SW/Engine/System Instance 1/HCI [1,..,n] ==
  Switch : Constant  Value=CPT.MDL_SW.Engine{1}.HCI.Switch.v
  Terminator : Terminator
  tag scope: Engine_1_HCI_SW=global
  wires:
  [Engine_1_HCI_SW] -> Terminator/1
  Switch/1 -> [Engine_1_HCI_SW]

== system Demo_veDYNA_cs/Vedyna_Vehicle/CPT_MDL/MDL_SW/Engine/System Instance 1/MSR_Flag [1,..,4] ==
  Switch : Constant  Value=CPT.MDL_SW.Engine{1}.MSR_Flag.Switch.v
  Terminator : Terminator
  tag scope: Engine_1_MSR_Flag_SW=global
  wires:
  [Engine_1_MSR_Flag_SW] -> Terminator/1
  Switch/1 -> [Engine_1_MSR_Flag_SW]

== system Demo_veDYNA_cs/Vedyna_Vehicle/CPT_MDL/MDL_SW/Engine/System Instance 1/MSR_Torque [1,..,4] ==
  Switch : Constant  Value=CPT.MDL_SW.Engine{1}.MSR_Torque.Switch.v
  Terminator : Terminator
  tag scope: Engine_1_MSR_Torque_SW=global
  wires:
  [Engine_1_MSR_Torque_SW] -> Terminator/1
  Switch/1 -> [Engine_1_MSR_Torque_SW]

== system Demo_veDYNA_cs/Vedyna_Vehicle/CPT_MDL/MDL_SW/GearCtrl/System Instance 1/Gear [1,..,4] ==
  Switch : Constant  Value=CPT.MDL_SW.GearCtrl{1}.Gear.Switch.v
  Terminator : Terminator
  tag scope: GearCtrl_1_Gear_SW=global
  wires:
  [GearCtrl_1_Gear_SW] -> Terminator/1
  Switch/1 -> [GearCtrl_1_Gear_SW]

== system Demo_veDYNA_cs/Vedyna_Vehicle/CPT_MDL/MDL_SW/GearCtrl/System Instance 1/GearMode [0,1] ==
  Switch : Constant  Value=CPT.MDL_SW.GearCtrl{1}.GearMode.Switch.v
  Terminator : Terminator
  tag scope: GearCtrl_1_GearMode_SW=global
  wires:
  [GearCtrl_1_GearMode_SW] -> Terminator/1
  Switch/1 -> [GearCtrl_1_GearMode_SW]

== system Demo_veDYNA_cs/Vedyna_Vehicle/CPT_MDL/MDL_SW/GearCtrl/System Instance 1/HCI [1,..,n] ==
  Switch : Constant  Value=CPT.MDL_SW.GearCtrl{1}.HCI.Switch.v
  Terminator : Terminator
  tag scope: GearCtrl_1_HCI_SW=global
  wires:
  [GearCtrl_1_HCI_SW] -> Terminator/1
  Switch/1 -> [GearCtrl_1_HCI_SW]

== system Demo_veDYNA_cs/Vedyna_Vehicle/CPT_MDL/MDL_SW/GearCtrl/System Instance 1/UpShiftRequest [1,..,4] ==
  Switch : Constant  Value=CPT.MDL_SW.GearCtrl{1}.UpShiftRequest.Switch.v
  Terminator : Terminator
  tag scope: GearCtrl_1_UpShiftRequest_SW=global
  wires:
  [GearCtrl_1_UpShiftRequest_SW] -> Terminator/1
  Switch/1 -> [GearCtrl_1_UpShiftRequest_SW]

== system Demo_veDYNA_cs/Vedyna_Vehicle/CPT_MDL/MDL_SW/ManLatCtrl/System Instance 1/Curvature [1,..,4] ==
  Switch : Constant  Value=CPT.MDL_SW.ManLatCtrl{1}.Curvature.Switch.v
  Terminator : Terminator
  tag scope: ManLatCtrl_1_Curvature_SW=global
  wires:
  [ManLatCtrl_1_Curvature_SW] -> Terminator/1
  Switch/1 -> [ManLatCtrl_1_Curvature_SW]

== system Demo_veDYNA_cs/Vedyna_Vehicle/CPT_MDL/MDL_SW/ManLatCtrl/System Instance 1/LatManMode [0,1,2] ==
  Switch : Constant  Value=CPT.MDL_SW.ManLatCtrl{1}.LatManMode.Switch.v
  Terminator : Terminator
  tag scope: ManLatCtrl_1_LatManMode_SW=global
  wires:
  [ManLatCtrl_1_LatManMode_SW] -> Terminator/1
  Switch/1 -> [ManLatCtrl_1_LatManMode_SW]

== system Demo_veDYNA_cs/Vedyna_Vehicle/CPT_MDL/MDL_SW/ManLatCtrl/System Instance 1/Steering [1,..,4] ==
  Switch : Constant  Value=CPT.MDL_SW.ManLatCtrl{1}.Steering.Switch.v
  Terminator : Terminator
  tag scope: ManLatCtrl_1_Steering_SW=global
  wires:
  [ManLatCtrl_1_Steering_SW] -> Terminator/1
  Switch/1 -> [ManLatCtrl_1_Steering_SW]

== system Demo_veDYNA_cs/Vedyna_Vehicle/CPT_MDL/MDL_SW/ManLongCtrl/System Instance 1/AccelerationY [1,..,4] ==
  Switch : Constant  Value=CPT.MDL_SW.ManLongCtrl{1}.AccelerationY.Switch.v
  Terminator : Terminator
  tag scope: ManLongCtrl_1_AccelerationY_SW=global
  wires:
  [ManLongCtrl_1_AccelerationY_SW] -> Terminator/1
  Switch/1 -> [ManLongCtrl_1_AccelerationY_SW]

== system Demo_veDYNA_cs/Vedyna_Vehicle/CPT_MDL/MDL_SW/ManLongCtrl/System Instance 1/Brake [1,..,4] ==
  Switch : Constant  Value=CPT.MDL_SW.ManLongCtrl{1}.Brake.Switch.v
  Terminator : Terminator
  tag scope: ManLongCtrl_1_Brake_SW=global
  wires:
  [ManLongCtrl_1_Brake_SW] -> Terminator/1
  Switch/1 -> [ManLongCtrl_1_Brake_SW]

== system Demo_veDYNA_cs/Vedyna_Vehicle/CPT_MDL/MDL_SW/ManLongCtrl/System Instance 1/EngineTorque [1,..,4] ==
  Switch : Constant  Value=CPT.MDL_SW.ManLongCtrl{1}.EngineTorque.Switch.v
  Terminator : Terminator
  tag scope: ManLongCtrl_1_EngineTorque_SW=global
  wires:
  [ManLongCtrl_1_EngineTorque_SW] -> Terminator/1
  Switch/1 -> [ManLongCtrl_1_EngineTorque_SW]

== system Demo_veDYNA_cs/Vedyna_Vehicle/CPT_MDL/MDL_SW/ManLongCtrl/System Instance 1/LongManMode [0,1,2] ==
  Switch : Constant  Value=CPT.MDL_SW.ManLongCtrl{1}.LongManMode.Switch.v
  Terminator : Terminator
  tag scope: ManLongCtrl_1_LongManMode_SW=global
  wires:
  [ManLongCtrl_1_LongManMode_SW] -> Terminator/1
  Switch/1 -> [ManLongCtrl_1_LongManMode_SW]

== system Demo_veDYNA_cs/Vedyna_Vehicle/CPT_MDL/MDL_SW/ManLongCtrl/System Instance 1/Speed [1,..,4] ==
  Switch : Constant  Value=CPT.MDL_SW.ManLongCtrl{1}.Speed.Switch.v
  Terminator : Terminator
  tag scope: ManLongCtrl_1_Speed_SW=global
  wires:
  [ManLongCtrl_1_Speed_SW] -> Terminator/1
  Switch/1 -> [ManLongCtrl_1_Speed_SW]

== system Demo_veDYNA_cs/Vedyna_Vehicle/CPT_MDL/MDL_SW/ManLongCtrl/System Instance 1/Throttle [1,..,4] ==
  Switch : Constant  Value=CPT.MDL_SW.ManLongCtrl{1}.Throttle.Switch.v
  Terminator : Terminator
  tag scope: ManLongCtrl_1_Throttle_SW=global
  wires:
  [ManLongCtrl_1_Throttle_SW] -> Terminator/1
  Switch/1 -> [ManLongCtrl_1_Throttle_SW]

== system Demo_veDYNA_cs/Vedyna_Vehicle/CPT_MDL/MDL_SW/ManSchedule/System Instance 1/HCI [1,..,n] ==
  Switch : Constant  Value=CPT.MDL_SW.ManSchedule{1}.HCI.Switch.v
  Terminator : Terminator
  tag scope: ManSchedule_1_HCI_SW=global
  wires:
  [ManSchedule_1_HCI_SW] -> Terminator/1
  Switch/1 -> [ManSchedule_1_HCI_SW]

== system Demo_veDYNA_cs/Vedyna_Vehicle/CPT_MDL/MDL_SW/ManSchedule/System Instance 2/HCI [1,..,n] ==
  Switch : Constant  Value=CPT.MDL_SW.ManSchedule{2}.HCI.Switch.v
  Terminator : Terminator
  tag scope: ManSchedule_2_HCI_SW=global
  wires:
  [ManSchedule_2_HCI_SW] -> Terminator/1
  Switch/1 -> [ManSchedule_2_HCI_SW]

== system Demo_veDYNA_cs/Vedyna_Vehicle/CPT_MDL/MDL_SW/ManSchedule/System Instance 3/HCI [1,..,n] ==
  Switch : Constant  Value=CPT.MDL_SW.ManSchedule{3}.HCI.Switch.v
  Terminator : Terminator
  tag scope: ManSchedule_3_HCI_SW=global
  wires:
  [ManSchedule_3_HCI_SW] -> Terminator/1
  Switch/1 -> [ManSchedule_3_HCI_SW]

== system Demo_veDYNA_cs/Vedyna_Vehicle/CPT_MDL/MDL_SW/Road/System Instance 1/HCI [1,..,n] ==
  Switch : Constant  Value=CPT.MDL_SW.Road{1}.HCI.Switch.v
  Terminator : Terminator
  tag scope: Road_1_HCI_SW=global
  wires:
  [Road_1_HCI_SW] -> Terminator/1
  Switch/1 -> [Road_1_HCI_SW]

== system Demo_veDYNA_cs/Vedyna_Vehicle/CPT_MDL/MDL_SW/Simctrl/System Instance 1/Reset [0,1] ==
  Switch : Constant  Value=CPT.MDL_SW.Simctrl{1}.Reset.Switch.v
  Terminator : Terminator
  tag scope: Simctrl_1_Reset_SW=global
  wires:
  [Simctrl_1_Reset_SW] -> Terminator/1
  Switch/1 -> [Simctrl_1_Reset_SW]

== system Demo_veDYNA_cs/Vedyna_Vehicle/CPT_MDL/MDL_SW/Simctrl/System Instance 1/Suspend [0,1] ==
  Switch : Constant  Value=CPT.MDL_SW.Simctrl{1}.Suspend.Switch.v
  Terminator : Terminator
  tag scope: Simctrl_1_Suspend_SW=global
  wires:
  [Simctrl_1_Suspend_SW] -> Terminator/1
  Switch/1 -> [Simctrl_1_Suspend_SW]

== system Demo_veDYNA_cs/Vedyna_Vehicle/CPT_MDL/MDL_SW/Tmeasy/System Instance 1/HCI [1,..,n] ==
  Switch : Constant  Value=CPT.MDL_SW.Tmeasy{1}.HCI.Switch.v
  Terminator : Terminator
  tag scope: Tmeasy_1_HCI_SW=global
  wires:
  [Tmeasy_1_HCI_SW] -> Terminator/1
  Switch/1 -> [Tmeasy_1_HCI_SW]

== system Demo_veDYNA_cs/Vedyna_Vehicle/CPT_MDL/MDL_SW/Tmeasy/System Instance 1/RoadMueScale [1,..,4] ==
  Switch : Constant  Value=CPT.MDL_SW.Tmeasy{1}.RoadMueScale.Switch.v
  Terminator : Terminator
  tag scope: Tmeasy_1_RoadMueScale_SW=global
  wires:
  [Tmeasy_1_RoadMueScale_SW] -> Terminator/1
  Switch/1 -> [Tmeasy_1_RoadMueScale_SW]

== system Demo_veDYNA_cs/Vedyna_Vehicle/CPT_MDL/MDL_SW/Tmeasy/System Instance 2/HCI [1,..,n] ==
  Switch : Constant  Value=CPT.MDL_SW.Tmeasy{2}.HCI.Switch.v
  Terminator : Terminator
  tag scope: Tmeasy_2_HCI_SW=global
  wires:
  [Tmeasy_2_HCI_SW] -> Terminator/1
  Switch/1 -> [Tmeasy_2_HCI_SW]

== system Demo_veDYNA_cs/Vedyna_Vehicle/CPT_MDL/MDL_SW/Tmeasy/System Instance 2/RoadMueScale [1,..,4] ==
  Switch : Constant  Value=CPT.MDL_SW.Tmeasy{2}.RoadMueScale.Switch.v
  Terminator : Terminator
  tag scope: Tmeasy_2_RoadMueScale_SW=global
  wires:
  [Tmeasy_2_RoadMueScale_SW] -> Terminator/1
  Switch/1 -> [Tmeasy_2_RoadMueScale_SW]

== system Demo_veDYNA_cs/Vedyna_Vehicle/CPT_MDL/MDL_SW/Tmeasy/System Instance 3/HCI [1,..,n] ==
  Switch : Constant  Value=CPT.MDL_SW.Tmeasy{3}.HCI.Switch.v
  Terminator : Terminator
  tag scope: Tmeasy_3_HCI_SW=global
  wires:
  [Tmeasy_3_HCI_SW] -> Terminator/1
  Switch/1 -> [Tmeasy_3_HCI_SW]

== system Demo_veDYNA_cs/Vedyna_Vehicle/CPT_MDL/MDL_SW/Tmeasy/System Instance 3/RoadMueScale [1,..,4] ==
  Switch : Constant  Value=CPT.MDL_SW.Tmeasy{3}.RoadMueScale.Switch.v
  Terminator : Terminator
  tag scope: Tmeasy_3_RoadMueScale_SW=global
  wires:
  [Tmeasy_3_RoadMueScale_SW] -> Terminator/1
  Switch/1 -> [Tmeasy_3_RoadMueScale_SW]

== system Demo_veDYNA_cs/Vedyna_Vehicle/CPT_MDL/MDL_SW/Tmeasy/System Instance 4/HCI [1,..,n] ==
  Switch : Constant  Value=CPT.MDL_SW.Tmeasy{4}.HCI.Switch.v
  Terminator : Terminator
  tag scope: Tmeasy_4_HCI_SW=global
  wires:
  [Tmeasy_4_HCI_SW] -> Terminator/1
  Switch/1 -> [Tmeasy_4_HCI_SW]

== system Demo_veDYNA_cs/Vedyna_Vehicle/CPT_MDL/MDL_SW/Tmeasy/System Instance 4/RoadMueScale [1,..,4] ==
  Switch : Constant  Value=CPT.MDL_SW.Tmeasy{4}.RoadMueScale.Switch.v
  Terminator : Terminator
  tag scope: Tmeasy_4_RoadMueScale_SW=global
  wires:
  [Tmeasy_4_RoadMueScale_SW] -> Terminator/1
  Switch/1 -> [Tmeasy_4_RoadMueScale_SW]

== system Demo_veDYNA_cs/Vedyna_Vehicle/CPT_MDL/MDL_SW/Tmeasy/System Instance 5/HCI [1,..,n] ==
  Switch : Constant  Value=CPT.MDL_SW.Tmeasy{5}.HCI.Switch.v
  Terminator : Terminator
  tag scope: Tmeasy_5_HCI_SW=global
  wires:
  [Tmeasy_5_HCI_SW] -> Terminator/1
  Switch/1 -> [Tmeasy_5_HCI_SW]

== system Demo_veDYNA_cs/Vedyna_Vehicle/CPT_MDL/MDL_SW/Tmeasy/System Instance 5/RoadMueScale [1,..,4] ==
  Switch : Constant  Value=CPT.MDL_SW.Tmeasy{5}.RoadMueScale.Switch.v
  Terminator : Terminator
  tag scope: Tmeasy_5_RoadMueScale_SW=global
  wires:
  [Tmeasy_5_RoadMueScale_SW] -> Terminator/1
  Switch/1 -> [Tmeasy_5_RoadMueScale_SW]

== system Demo_veDYNA_cs/Vedyna_Vehicle/CPT_MDL/MDL_SW/Tmeasy/System Instance 6/HCI [1,..,n] ==
  Switch : Constant  Value=CPT.MDL_SW.Tmeasy{6}.HCI.Switch.v
  Terminator : Terminator
  tag scope: Tmeasy_6_HCI_SW=global
  wires:
  [Tmeasy_6_HCI_SW] -> Terminator/1
  Switch/1 -> [Tmeasy_6_HCI_SW]

== system Demo_veDYNA_cs/Vedyna_Vehicle/CPT_MDL/MDL_SW/Tmeasy/System Instance 6/RoadMueScale [1,..,4] ==
  Switch : Constant  Value=CPT.MDL_SW.Tmeasy{6}.RoadMueScale.Switch.v
  Terminator : Terminator
  tag scope: Tmeasy_6_RoadMueScale_SW=global
  wires:
  [Tmeasy_6_RoadMueScale_SW] -> Terminator/1
  Switch/1 -> [Tmeasy_6_RoadMueScale_SW]

== system Demo_veDYNA_cs/Vedyna_Vehicle/CPT_MDL/MDL_SW/Tmeasy/System Instance 7/HCI [1,..,n] ==
  Switch : Constant  Value=CPT.MDL_SW.Tmeasy{7}.HCI.Switch.v
  Terminator : Terminator
  tag scope: Tmeasy_7_HCI_SW=global
  wires:
  Switch/1 -> [Tmeasy_7_HCI_SW]
  [Tmeasy_7_HCI_SW] -> Terminator/1

== system Demo_veDYNA_cs/Vedyna_Vehicle/CPT_MDL/MDL_SW/Tmeasy/System Instance 7/RoadMueScale [1,..,4] ==
  Switch : Constant  Value=CPT.MDL_SW.Tmeasy{7}.RoadMueScale.Switch.v
  Terminator : Terminator
  tag scope: Tmeasy_7_RoadMueScale_SW=global
  wires:
  Switch/1 -> [Tmeasy_7_RoadMueScale_SW]
  [Tmeasy_7_RoadMueScale_SW] -> Terminator/1

== system Demo_veDYNA_cs/Vedyna_Vehicle/CPT_MDL/MDL_SW/Tmeasy/System Instance 8/HCI [1,..,n] ==
  Switch : Constant  Value=CPT.MDL_SW.Tmeasy{8}.HCI.Switch.v
  Terminator : Terminator
  tag scope: Tmeasy_8_HCI_SW=global
  wires:
  Switch/1 -> [Tmeasy_8_HCI_SW]
  [Tmeasy_8_HCI_SW] -> Terminator/1

== system Demo_veDYNA_cs/Vedyna_Vehicle/CPT_MDL/MDL_SW/Tmeasy/System Instance 8/RoadMueScale [1,..,4] ==
  Switch : Constant  Value=CPT.MDL_SW.Tmeasy{8}.RoadMueScale.Switch.v
  Terminator : Terminator
  tag scope: Tmeasy_8_RoadMueScale_SW=global
  wires:
  Switch/1 -> [Tmeasy_8_RoadMueScale_SW]
  [Tmeasy_8_RoadMueScale_SW] -> Terminator/1

== system Demo_veDYNA_cs/Vedyna_Vehicle/CPT_MDL/MDL_SW/Vehicle/System Instance 1/HCI [1,..,n] ==
  Switch : Constant  Value=CPT.MDL_SW.Vehicle{1}.HCI.Switch.v
  Terminator : Terminator
  tag scope: Vehicle_1_HCI_SW=global
  wires:
  [Vehicle_1_HCI_SW] -> Terminator/1
  Switch/1 -> [Vehicle_1_HCI_SW]

== system Demo_veDYNA_cs/Vedyna_Vehicle/CPT_MDL/MDL_SW/Wheel/System Instance 1/HCI [1,..,n] ==
  Switch : Constant  Value=CPT.MDL_SW.Wheel{1}.HCI.Switch.v
  Terminator : Terminator
  tag scope: Wheel_1_HCI_SW=global
  wires:
  [Wheel_1_HCI_SW] -> Terminator/1
  Switch/1 -> [Wheel_1_HCI_SW]

== system Demo_veDYNA_cs/Vedyna_Vehicle/CPT_MDL/MDL_SW/Wheel/System Instance 1/pbrm [1,..,4] ==
  Switch : Constant  Value=CPT.MDL_SW.Wheel{1}.pbrm.Switch.v
  Terminator : Terminator
  tag scope: Wheel_1_pbrm_SW=global
  wires:
  [Wheel_1_pbrm_SW] -> Terminator/1
  Switch/1 -> [Wheel_1_pbrm_SW]

== system Demo_veDYNA_cs/Vedyna_Vehicle/CPT_MDL/MDL_SW/Wheel/System Instance 2/HCI [1,..,n] ==
  Switch : Constant  Value=CPT.MDL_SW.Wheel{2}.HCI.Switch.v
  Terminator : Terminator
  tag scope: Wheel_2_HCI_SW=global
  wires:
  [Wheel_2_HCI_SW] -> Terminator/1
  Switch/1 -> [Wheel_2_HCI_SW]

== system Demo_veDYNA_cs/Vedyna_Vehicle/CPT_MDL/MDL_SW/Wheel/System Instance 2/pbrm [1,..,4] ==
  Switch : Constant  Value=CPT.MDL_SW.Wheel{2}.pbrm.Switch.v
  Terminator : Terminator
  tag scope: Wheel_2_pbrm_SW=global
  wires:
  [Wheel_2_pbrm_SW] -> Terminator/1
  Switch/1 -> [Wheel_2_pbrm_SW]

== system Demo_veDYNA_cs/Vedyna_Vehicle/CPT_MDL/MDL_SW/Wheel/System Instance 3/HCI [1,..,n] ==
  Switch : Constant  Value=CPT.MDL_SW.Wheel{3}.HCI.Switch.v
  Terminator : Terminator
  tag scope: Wheel_3_HCI_SW=global
  wires:
  [Wheel_3_HCI_SW] -> Terminator/1
  Switch/1 -> [Wheel_3_HCI_SW]

== system Demo_veDYNA_cs/Vedyna_Vehicle/CPT_MDL/MDL_SW/Wheel/System Instance 3/pbrm [1,..,4] ==
  Switch : Constant  Value=CPT.MDL_SW.Wheel{3}.pbrm.Switch.v
  Terminator : Terminator
  tag scope: Wheel_3_pbrm_SW=global
  wires:
  [Wheel_3_pbrm_SW] -> Terminator/1
  Switch/1 -> [Wheel_3_pbrm_SW]

== system Demo_veDYNA_cs/Vedyna_Vehicle/CPT_MDL/MDL_SW/Wheel/System Instance 4/HCI [1,..,n] ==
  Switch : Constant  Value=CPT.MDL_SW.Wheel{4}.HCI.Switch.v
  Terminator : Terminator
  tag scope: Wheel_4_HCI_SW=global
  wires:
  [Wheel_4_HCI_SW] -> Terminator/1
  Switch/1 -> [Wheel_4_HCI_SW]

== system Demo_veDYNA_cs/Vedyna_Vehicle/CPT_MDL/MDL_SW/Wheel/System Instance 4/pbrm [1,..,4] ==
  Switch : Constant  Value=CPT.MDL_SW.Wheel{4}.pbrm.Switch.v
  Terminator : Terminator
  tag scope: Wheel_4_pbrm_SW=global
  wires:
  [Wheel_4_pbrm_SW] -> Terminator/1
  Switch/1 -> [Wheel_4_pbrm_SW]

== system Demo_veDYNA_cs/Vedyna_Vehicle/CPT_MDL/MDL_SW/Wheel/System Instance 5/HCI [1,..,n] ==
  Switch : Constant  Value=CPT.MDL_SW.Wheel{5}.HCI.Switch.v
  Terminator : Terminator
  tag scope: Wheel_5_HCI_SW=global
  wires:
  [Wheel_5_HCI_SW] -> Terminator/1
  Switch/1 -> [Wheel_5_HCI_SW]

== system Demo_veDYNA_cs/Vedyna_Vehicle/CPT_MDL/MDL_SW/Wheel/System Instance 5/pbrm [1,..,4] ==
  Switch : Constant  Value=CPT.MDL_SW.Wheel{5}.pbrm.Switch.v
  Terminator : Terminator
  tag scope: Wheel_5_pbrm_SW=global
  wires:
  [Wheel_5_pbrm_SW] -> Terminator/1
  Switch/1 -> [Wheel_5_pbrm_SW]

== system Demo_veDYNA_cs/Vedyna_Vehicle/CPT_MDL/MDL_SW/Wheel/System Instance 6/HCI [1,..,n] ==
  Switch : Constant  Value=CPT.MDL_SW.Wheel{6}.HCI.Switch.v
  Terminator : Terminator
  tag scope: Wheel_6_HCI_SW=global
  wires:
  [Wheel_6_HCI_SW] -> Terminator/1
  Switch/1 -> [Wheel_6_HCI_SW]

== system Demo_veDYNA_cs/Vedyna_Vehicle/CPT_MDL/MDL_SW/Wheel/System Instance 6/pbrm [1,..,4] ==
  Switch : Constant  Value=CPT.MDL_SW.Wheel{6}.pbrm.Switch.v
  Terminator : Terminator
  tag scope: Wheel_6_pbrm_SW=global
  wires:
  [Wheel_6_pbrm_SW] -> Terminator/1
  Switch/1 -> [Wheel_6_pbrm_SW]
